simulink model "wo_buckswitch"  (R2016a)
settings: Solver=ode23tb  StartTime=0.0  StopTime=0.1  RelTol=1e-6
undefined symbols (not defined in the file or in its folder): Vc_bat
libraries: powerlib x12, simulink x2
settings Model: Creator=mugino  LastModifiedBy=mugino
settings SolverCC: AlgebraicLoopSolver=LineSearch
settings DebuggingCC: IgnoredZcDiagnostic=none

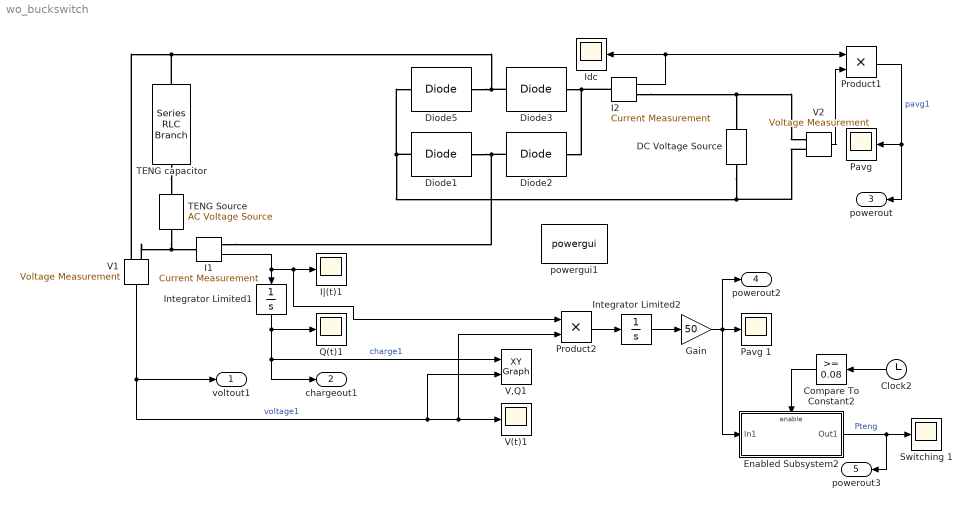
== system wo_buckswitch ==
  Clock2 : Clock
  Compare To Constant2 : simulink/Logic and Bit Operations/Compare To Constant  relop=>=  const=0.08  OutDataTypeStr=boolean
  DC Voltage Source : powerlib/Electrical Sources/DC Voltage Source  Amplitude=Vc_bat  Measurements=None
  Diode{1..3,5} (4 alike) : powerlib/Power Electronics/Diode  Ron=0.01  Lon=1e-3  Vf=0.7  IC=0  UseSnubber=off  Rs=500  Cs=6e-12  Measurements=off
  Enabled Subsystem2 : Subsystem  TreatAsAtomicUnit=on
  Gain : Gain  Gain=50
  I1 : powerlib/Measurements/Current Measurement  PhasorSimulation=off  OutputType=Complex  PSBequivalent=0
  I2 : powerlib/Measurements/Current Measurement  PhasorSimulation=off  OutputType=Complex  PSBequivalent=0
  Idc : Scope
  Integrator Limited1 : Integrator  LimitOutput=on  UpperSaturationLimit=1  LowerSaturationLimit=0
  Integrator Limited2 : Integrator  LimitOutput=on  UpperSaturationLimit=10  LowerSaturationLimit=0  IgnoreLimit=on
  I|(t)1 : Scope
  "Pavg " : Scope
  Pavg 1 : Scope
  Product1 : Product
  Product2 : Product
  Q(t)1 : Scope
  Switching 1 : Scope
  TENG Source : powerlib/Electrical Sources/AC Voltage Source  Amplitude=150  Phase=0  Frequency=50  SampleTime=0  Measurements=None  BusType=PV  Pref=10e3  Qref=0  Qmin=-inf  Qmax=+inf
  TENG capacitor : powerlib/Elements/Series RLC Branch  LConnTagsString=__new0  RConnTagsString=__new0  BranchType=RC  Resistance=1000  Inductance=1e-3  SetiL0=off  InitialCurrent=0  Capacitance=1.5e-10  Setx0=off  InitialVoltage=0  Measurements=None
  V(t)1 : Scope
  V,Q1 : simulink/Sinks/XY Graph  xmin=-1e-9  xmax=50e-9  ymin=-150  ymax=150  st=-1
  V1 : powerlib/Measurements/Voltage Measurement  PhasorSimulation=off  OutputType=Complex  PSBequivalent=0
  V2 : powerlib/Measurements/Voltage Measurement  PhasorSimulation=off  OutputType=Complex  PSBequivalent=0
  powergui1 : powerlib/powergui  Priority=1  SimulationMode=Continuous  SolverType=Tustin/Backward Euler (TBE)  SampleTime=50e-6  frequency=60  SPID=on  DisableSnubberDevices=off  DisableRonSwitches=off  DisableVfSwitches=off  SwTol=0  DisplayEquations=off  Interpol=off  ExternalGateDelay=off  methode=off  Ts=10  FunctionMessages=off  echomessages=off  HookPort=off  EnableUseOfTLC=off  x0status=steady  frequencyindice=0  Pbase=100e6  ErrMax=1e-4  Iterations=50  UnitsV=kV  UnitsW=MW  buscounter=0  RestoreLinks=warning  ResistiveCurrentMeasurement=off  Frange=[0:2:500]  Ylog=off  Xlog=on  ShowGrid=off  save=off  variable=ZData  structure=0  ZoomFFT=off  StartTime=0.0  cycles=1  DisplayStyle=1  fundamental=60  FreqAxis=off  MaxFrequency=1000  frequencyindicesteady=1  RmsSteady=2  display=off
  voltout1 : Outport
  chargeout1 : Outport  Port=2
  powerout : Outport  Port=3
  powerout2 : Outport  Port=4
  powerout3 : Outport  Port=5
  wires:
  Integrator Limited1/1 -> chargeout1/1, V,Q1/1, Q(t)1/1  "charge1"
  V1/1 -> voltout1/1, V,Q1/2, Product2/2, V(t)1/1  "voltage1"
  I1/1 -> Integrator Limited1/1, Product2/1, I|(t)1/1
  V2/1 -> Product1/2
  Product1/1 -> "Pavg "/1, powerout/1  "pavg1"
  I2/1 -> Idc/1, Product1/1
  Product2/1 -> Integrator Limited2/1
  Integrator Limited2/1 -> Gain/1
  Gain/1 -> Enabled Subsystem2/1(In1), powerout2/1, Pavg 1/1
  Compare To Constant2/1 -> Enabled Subsystem2/Enable
  Enabled Subsystem2/1(Out1) -> powerout3/1, Switching 1/1  "Pteng"
  Clock2/1 -> Compare To Constant2/1
  connections:
  V1/LConn1 -- Diode3/LConn1 -- Diode5/RConn1 -- TENG capacitor/LConn1
  I1/RConn1 -- Diode2/LConn1 -- Diode1/RConn1
  I2/LConn1 -- Diode3/RConn1 -- Diode2/RConn1
  V1/LConn2 -- TENG Source/LConn1 -- I1/LConn1
  Diode5/LConn1 -- Diode1/LConn1 -- V2/LConn2 -- DC Voltage Source/LConn1
  TENG capacitor/RConn1 -- TENG Source/RConn1
  I2/RConn1 -- DC Voltage Source/RConn1 -- V2/LConn1

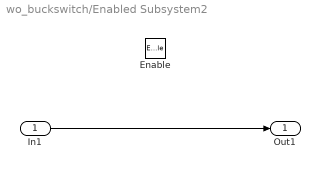
== system wo_buckswitch/Enabled Subsystem2 ==
  In1 : Inport
  Enable : EnablePort
  Out1 : Outport
  wires:
  In1/1 -> Out1/1
